simulink model "EMPlanner_850_155633_cs"  (R2023a)
settings: Solver=ode5  StartTime=0.0  StopTime=30  FixedStep=1/1000  RelTol=1e-3
PreLoadFcn:
  | mbxruntime.callbacks.PreLoadFcn(bdroot);
PostLoadFcn:
  | mbxruntime.callbacks.PostLoadFcn(bdroot);
InitFcn:
  | mbxruntime.callbacks.InitFcn(bdroot);
StartFcn:
  | mbxruntime.callbacks.StartFcn(bdroot);
StopFcn:
  | mbxruntime.callbacks.StopFcn(bdroot);
model workspace (MAT data in the model file):
  mbox_table : object (value not decoded)
  model_closed = 0
  sim_status = 0
undefined symbols (not defined in the file): aubr, c_factor, cf, cr, DiscIntNeverNeededParam, global_path_x, global_path_y, KD_PID_distance, KD_PID_speed, KI_PID_distance, KI_PID_speed, KP_PID_distance, KP_PID_speed, la, lb, LQR_K1, LQR_K2, LQR_K3, LQR_K4, m, rack_displacement, right_wheel_ground, tablebr, vubr, vx_break_point, warningInitialVelocity, x0
libraries: PreScanSimulinkLibrary x39, simulink x19, simulink_extras x11, Solver_SF x1
(part 9 of 11)

== matlab function EMPlanner_850_155633_cs/Audi_A8_Sedan_1/decision&planning module/referenceline provider/MATLAB Function5 ==
  data: x_set input; match_point_index_set output; y_set input; frenet_path_x input; frenet_path_y input; frenet_path_heading input; frenet_path_kappa input; proj_x_set output; proj_y_set output; proj_heading_set output; proj_kappa_set output
function [match_point_index_set,proj_x_set, proj_y_set,proj_heading_set,proj_kappa_set] = ...
    fcn(x_set,y_set,frenet_path_x,frenet_path_y,frenet_path_heading,frenet_path_kappa)
%该函数将批量计算x_set，y_set中的xy，在frenet_path下的投影的信息
%输入 x_set,y_set，待投影的点的集合
%x_set,y_set,frenet_path_x,frenet_path_y,frenet_path_heading,frenet_path_kappa
%曲线在直角坐标系下的x，y，heading，kappa
%输出：match_point_index_set 匹配点在frenet_path下的编号的集合(即从全局路径第一个点开始数，第几个点是匹配点)
%     proj_x y heading kappa 投影的x,y,heading,kappa的集合

% 由于事先不知道x_set中到底有多少个点需要投影，因此事先声明一个最大的数量的点作为缓冲
n = 128;
% 并且由于不知道投影点的个数，所以也不知道输出的个数，因此输出也要做缓冲，用nan表示不存在的点
% 输出最多输出128个
% 输出初始化
match_point_index_set = ones(n,1) * nan;
proj_x_set = ones(n,1) * nan;
proj_y_set = ones(n,1) * nan;
proj_heading_set = ones(n,1) * nan;
proj_kappa_set = ones(n,1) * nan;

% 找匹配点，需要利用上一个周期的结果作为下一个周期遍历的起点，因此需要声明两个全局变量

persistent is_first_run;
persistent pre_match_point_index_set;%bug :pre_match_point_index(i) 未必代表的是第i个障碍物的match_point_index
persistent pre_frenet_path_x;
persistent pre_frenet_path_y;
persistent pre_frenet_path_heading;
persistent pre_frenet_path_kappa;
persistent pre_x_set;
persistent pre_y_set;
%算法主函数入口

if isempty(is_first_run)
    %该if分支表示函数首次运行
    is_first_run = 0;
    pre_frenet_path_x = frenet_path_x;
    pre_frenet_path_y = frenet_path_y;
    pre_frenet_path_heading = frenet_path_heading;
    pre_frenet_path_kappa = frenet_path_kappa;
    %要记录首次运行计算的匹配点的结果供下个周期运行，先初始化
    pre_match_point_index_set = ones(n,1) * nan;
    %对x_set,y_set的点做遍历，找到他们的匹配点
    for i = 1 : length(x_set)
        if isnan(x_set(i))
            break;
        end
        %首次运行时，没有任何提示，只能从frenet path的第一个点开始找
        start_search_index = 1;
        % 声明increase_count，用于表示在遍历时distance连续增加的个数
        increase_count = 0;
        % 开始遍历
        min_distance = inf;
        for j = start_search_index : length(frenet_path_x)
            distance = (x_set(i) - frenet_path_x(j))^2 + (y_set(i) - frenet_path_y(j))^2;
            if distance < min_distance
                min_distance = distance;
                match_point_index_set(i) = j;
                increase_count = 0;
            else
                increase_count = increase_count + 1;
            end
            %如果distance连续增加50次就不要再遍历了，节省时间
            if increase_count > 50
                break;
            end
        end
        
        %如何通过匹配点计算投影点，请参见《自动驾驶控制算法第七讲》
        %或《自动驾驶决策规划算法》第一章第三节
        
        %取出匹配点的编号
        match_point_index = match_point_index_set(i);
        %取出匹配点的信息
        match_point_x = frenet_path_x(match_point_index);
        match_point_y = frenet_path_y(match_point_index);
        match_point_heading = frenet_path_heading(match_point_index);
        match_point_kappa = frenet_path_kappa(match_point_index);
        %计算匹配点的方向向量与法向量
        vector_match_point = [match_point_x;match_point_y];
        vector_match_point_direction = [cos(match_point_heading);sin(match_point_heading)];
        %声明待投影点的位矢
        vector_r = [x_set(i);y_set(i)];
        
       %通过匹配点计算投影点
       vector_d = vector_r - vector_match_point;
       ds = vector_d' * vector_match_point_direction;
       vector_proj_point = vector_match_point + ds * vector_match_point_direction;
       proj_heading = match_point_heading + match_point_kappa * ds;
       proj_kappa = match_point_kappa;
       %计算结果输出
       proj_x_set(i) = vector_proj_point(1);
       proj_y_set(i) = vector_proj_point(2);
       proj_heading_set(i) = proj_heading;
       proj_kappa_set(i) = proj_kappa;
    end
    %匹配点的计算结果保存，供下一个周期使用
    pre_match_point_index_set = match_point_index_set;
    pre_x_set = x_set;
    pre_y_set = y_set;
else
    %此if分支表示不是首次运行
    %对每个x_set上的点做处理
    for i = 1 : length(x_set)
        %不是首次运行，对于点x_set(i),y_set(i)来说,start_search_index =
        %pre_match_point_index_set(i)
        start_search_index = pre_match_point_index_set(i);%上个周期匹配点的编号作为本周期搜索的起点
        % 判断帧与帧之间的障碍物是否为同一个
        square_dis = (x_set(i) - pre_x_set(i))^2 + (y_set(i) - pre_y_set(i))^2;
        if square_dis > 36
            % 帧与帧之间的物体的位置距离过大，认为是两个障碍物
            start_search_index = nan;
        end
        % 声明increase_count，用于表示在遍历时distance连续增加的个数
        %%%%%%%%%
        %对于障碍物检测而言，当感知第一次检测到障碍物时，算法并不是首次运行，此时 
        %pre_match_point_index_set的值是nan，如果还用上一时刻的结果作为本周期搜索的起点
        %必然会出问题，所以要修改
        % 声明increase_count_limit
        increase_count_limit = 5;
        if isnan(start_search_index)
            %没有上个周期的结果，那就不能只检查5次了
            increase_count_limit = 50;
            %搜索起点也要设为1
            start_search_index = 1;
        end
        increase_count = 0;
        % 开始遍历
        %这里多一个步骤，判断遍历的方向
        %计算上个周期匹配点的位矢
        vector_pre_match_point = [pre_frenet_path_x(start_search_index);pre_frenet_path_y(start_search_index)];
        vector_pre_match_point_direction = ...
            [cos(pre_frenet_path_heading(start_search_index));sin(pre_frenet_path_heading(start_search_index))];
        %判断遍历的方向
        flag = ([x_set(i);y_set(i)] - vector_pre_match_point)' * vector_pre_match_point_direction;
        min_distance = inf;
        if flag > 0.001
            for j = start_search_index : length(frenet_path_x)
                distance = (x_set(i) - frenet_path_x(j))^2 + (y_set(i) - frenet_path_y(j))^2;
                if distance < min_distance
                    min_distance = distance;
                    match_point_index_set(i) = j;
                    increase_count = 0;
                else
                    increase_count = increase_count + 1;
                end
                %如果distance连续增加increase_count_limit次就不要再遍历了，节省时间
                if increase_count > increase_count_limit
                    break;
                end
            end
        elseif flag < - 0.001
            for j = start_search_index : -1 : 1
                distance = (x_set(i) - frenet_path_x(j))^2 + (y_set(i) - frenet_path_y(j))^2;
                if distance < min_distance
                    min_distance = distance;
                    match_point_index_set(i) = j;
                    increase_count = 0;
                else
                    increase_count = increase_count + 1;
                end
                %如果distance连续增加increase_count_limit次就不要再遍历了，节省时间
                if increase_count > increase_count_limit
                    break;
                end
            end
        else
            match_point_index_set(i) = start_search_index;
        end
        
        %如何通过匹配点计算投影点，请参见《自动驾驶控制算法第七讲》
        %或《自动驾驶决策规划算法》第一章第三节
        
        %取出匹配点的编号
        match_point_index = match_point_index_set(i);
        %取出匹配点的信息
        match_point_x = frenet_path_x(match_point_index);
        match_point_y = frenet_path_y(match_point_index);
        match_point_heading = frenet_path_heading(match_point_index);
        match_point_kappa = frenet_path_kappa(match_point_index);
        %计算匹配点的方向向量与法向量
        vector_match_point = [match_point_x;match_point_y];
        vector_match_point_direction = [cos(match_point_heading);sin(match_point_heading)];
        %声明待投影点的位矢
        vector_r = [x_set(i);y_set(i)];
        
       %通过匹配点计算投影点
       vector_d = vector_r - vector_match_point;
       ds = vector_d' * vector_match_point_direction;
       vector_proj_point = vector_match_point + ds * vector_match_point_direction;
       proj_heading = match_point_heading + match_point_kappa * ds;
       proj_kappa = match_point_kappa;
       %计算结果输出
       proj_x_set(i) = vector_proj_point(1);
       proj_y_set(i) = vector_proj_point(2);
       proj_heading_set(i) = proj_heading;
       proj_kappa_set(i) = proj_kappa;
  
    end
    %匹配点的计算结果保存，供下一个周期使用
    pre_match_point_index_set = match_point_index_set;
    pre_frenet_path_x = frenet_path_x;
    pre_frenet_path_y = frenet_path_y;
    pre_frenet_path_heading = frenet_path_heading;
    pre_frenet_path_kappa = frenet_path_kappa;
    pre_x_set = x_set;
    pre_y_set = y_set;
end

== matlab function EMPlanner_850_155633_cs/Audi_A8_Sedan_1/decision&planning module/EM Planner/genrate index to s ==
  data: path_x input; index2s output; path_y input; origin_x input; origin_y input; origin_match_point_index input
function index2s  = fcn(path_x,path_y,origin_x,origin_y,origin_match_point_index)
%该函数将输出index与s的转换关系，index2s表示当path_x,path_y的离散点的编号为i时，对应的弧长为index2s(i)
%输入 path_x path_y 待转化的离散点的集合
%     origin_x,y frenet原点在世界坐标系下的坐标
%     origin_match_point_index 原点的匹配点的编号
% path点的个数
n = 181;
% 输出初始化
index2s = zeros(n,1);
% 首先计算以path起点为坐标原点的index2s
for i = 2:n
    index2s(i) = sqrt((path_x(i) - path_x(i-1))^2 + (path_y(i) - path_y(i-1))^2) + index2s(i-1);
end
% 再计算以轨迹起点到frenet_path的坐标原点的弧长，记为s0，再用index2s - s0 就是最终的结果
% 计算s0
% s_temp frenet原点的匹配点的弧长
s_temp = index2s(origin_match_point_index);
%判断原点在匹配点的前面还是后面
%两个向量match_point_to_origin 
%        match_point_to_match_point_next
vector_match_2_origin = [origin_x;origin_y] - [path_x(origin_match_point_index);path_y(origin_match_point_index)];
vector_match_2_match_next = [path_x(origin_match_point_index + 1);path_y(origin_match_point_index + 1)] - ...
                            [path_x(origin_match_point_index);path_y(origin_match_point_index)];
if vector_match_2_origin'*vector_match_2_match_next > 0
    %坐标原点在匹配点的前面
    s0 = s_temp + sqrt(vector_match_2_origin'*vector_match_2_origin);
else
    %坐标原点在匹配点的后面
    s0 = s_temp - sqrt(vector_match_2_origin'*vector_match_2_origin);
end

index2s = index2s - ones(n,1)*s0;

== stateflow chart EMPlanner_850_155633_cs/Audi_A8_Sedan_1/Chart ==
  (default) -> (junction 5)
  (junction 5) -> (junction 7)
  (junction 7) -> (junction 9) [order 1] : [i >= 100]
  (junction 7) -> (junction 13) [order 2] : {
      | i = i + 1;
      | }
  (junction 9) -> (junction 11) : {
      | do_planning;
      | i = 1;
      | }
  (junction 11) -> (junction 13)
  (junction 13) -> (junction 16)
  (junction 16) -> (junction 18) [order 1] : [j >= 10]
  (junction 16) -> (junction 22) [order 2] : {
      | j = j + 1;
      | }
  (junction 18) -> (junction 20) : {
      | do_control;
      | j = 1;
      | }
  (junction 20) -> (junction 22)
  (junction 22) -> (junction 25)
  data: i local =1; j local =1
  events: do_planning output FUNCTION_CALL_EVENT; do_control output FUNCTION_CALL_EVENT

== matlab function EMPlanner_850_155633_cs/Audi_A8_Sedan_1/decision&planning module/referenceline provider/MATLAB Function6 ==
  data: x_set input; match_point_index_set output; y_set input; frenet_path_x input; frenet_path_y input; frenet_path_heading input; frenet_path_kappa input; proj_x_set output; proj_y_set output; proj_heading_set output; proj_kappa_set output
function [match_point_index_set,proj_x_set, proj_y_set,proj_heading_set,proj_kappa_set] = ...
    fcn(x_set,y_set,frenet_path_x,frenet_path_y,frenet_path_heading,frenet_path_kappa)
%该函数将批量计算x_set，y_set中的xy，在frenet_path下的投影的信息
%输入 x_set,y_set，待投影的点的集合
%x_set,y_set,frenet_path_x,frenet_path_y,frenet_path_heading,frenet_path_kappa
%曲线在直角坐标系下的x，y，heading，kappa
%输出：match_point_index_set 匹配点在frenet_path下的编号的集合(即从全局路径第一个点开始数，第几个点是匹配点)
%     proj_x y heading kappa 投影的x,y,heading,kappa的集合

% 由于事先不知道x_set中到底有多少个点需要投影，因此事先声明一个最大的数量的点作为缓冲
n = 128;
% 并且由于不知道投影点的个数，所以也不知道输出的个数，因此输出也要做缓冲，用nan表示不存在的点
% 输出最多输出128个
% 输出初始化
match_point_index_set = ones(n,1) * nan;
proj_x_set = ones(n,1) * nan;
proj_y_set = ones(n,1) * nan;
proj_heading_set = ones(n,1) * nan;
proj_kappa_set = ones(n,1) * nan;

% 找匹配点，需要利用上一个周期的结果作为下一个周期遍历的起点，因此需要声明两个全局变量

persistent is_first_run;
persistent pre_match_point_index_set;%bug :pre_match_point_index(i) 未必代表的是第i个障碍物的match_point_index
persistent pre_frenet_path_x;
persistent pre_frenet_path_y;
persistent pre_frenet_path_heading;
persistent pre_frenet_path_kappa;
persistent pre_x_set;
persistent pre_y_set;
%算法主函数入口

if isempty(is_first_run)
    %该if分支表示函数首次运行
    is_first_run = 0;
    pre_frenet_path_x = frenet_path_x;
    pre_frenet_path_y = frenet_path_y;
    pre_frenet_path_heading = frenet_path_heading;
    pre_frenet_path_kappa = frenet_path_kappa;
    %要记录首次运行计算的匹配点的结果供下个周期运行，先初始化
    pre_match_point_index_set = ones(n,1) * nan;
    %对x_set,y_set的点做遍历，找到他们的匹配点
    for i = 1 : length(x_set)
        if isnan(x_set(i))
            break;
        end
        %首次运行时，没有任何提示，只能从frenet path的第一个点开始找
        start_search_index = 1;
        % 声明increase_count，用于表示在遍历时distance连续增加的个数
        increase_count = 0;
        % 开始遍历
        min_distance = inf;
        for j = start_search_index : length(frenet_path_x)
            distance = (x_set(i) - frenet_path_x(j))^2 + (y_set(i) - frenet_path_y(j))^2;
            if distance < min_distance
                min_distance = distance;
                match_point_index_set(i) = j;
                increase_count = 0;
            else
                increase_count = increase_count + 1;
            end
            %如果distance连续增加50次就不要再遍历了，节省时间
            if increase_count > 50
                break;
            end
        end
        
        %如何通过匹配点计算投影点，请参见《自动驾驶控制算法第七讲》
        %或《自动驾驶决策规划算法》第一章第三节
        
        %取出匹配点的编号
        match_point_index = match_point_index_set(i);
        %取出匹配点的信息
        match_point_x = frenet_path_x(match_point_index);
        match_point_y = frenet_path_y(match_point_index);
        match_point_heading = frenet_path_heading(match_point_index);
        match_point_kappa = frenet_path_kappa(match_point_index);
        %计算匹配点的方向向量与法向量
        vector_match_point = [match_point_x;match_point_y];
        vector_match_point_direction = [cos(match_point_heading);sin(match_point_heading)];
        %声明待投影点的位矢
        vector_r = [x_set(i);y_set(i)];
        
       %通过匹配点计算投影点
       vector_d = vector_r - vector_match_point;
       ds = vector_d' * vector_match_point_direction;
       vector_proj_point = vector_match_point + ds * vector_match_point_direction;
       proj_heading = match_point_heading + match_point_kappa * ds;
       proj_kappa = match_point_kappa;
       %计算结果输出
       proj_x_set(i) = vector_proj_point(1);
       proj_y_set(i) = vector_proj_point(2);
       proj_heading_set(i) = proj_heading;
       proj_kappa_set(i) = proj_kappa;
    end
    %匹配点的计算结果保存，供下一个周期使用
    pre_match_point_index_set = match_point_index_set;
    pre_x_set = x_set;
    pre_y_set = y_set;
else
    %此if分支表示不是首次运行
    %对每个x_set上的点做处理
    for i = 1 : length(x_set)
        %不是首次运行，对于点x_set(i),y_set(i)来说,start_search_index =
        %pre_match_point_index_set(i)
        start_search_index = pre_match_point_index_set(i);%上个周期匹配点的编号作为本周期搜索的起点
        % 判断帧与帧之间的障碍物是否为同一个
        square_dis = (x_set(i) - pre_x_set(i))^2 + (y_set(i) - pre_y_set(i))^2;
        if square_dis > 36
            % 帧与帧之间的物体的位置距离过大，认为是两个障碍物
            start_search_index = nan;
        end
        % 声明increase_count，用于表示在遍历时distance连续增加的个数
        %%%%%%%%%
        %对于障碍物检测而言，当感知第一次检测到障碍物时，算法并不是首次运行，此时 
        %pre_match_point_index_set的值是nan，如果还用上一时刻的结果作为本周期搜索的起点
        %必然会出问题，所以要修改
        % 声明increase_count_limit
        increase_count_limit = 5;
        if isnan(start_search_index)
            %没有上个周期的结果，那就不能只检查5次了
            increase_count_limit = 50;
            %搜索起点也要设为1
            start_search_index = 1;
        end
        increase_count = 0;
        % 开始遍历
        %这里多一个步骤，判断遍历的方向
        %计算上个周期匹配点的位矢
        vector_pre_match_point = [pre_frenet_path_x(start_search_index);pre_frenet_path_y(start_search_index)];
        vector_pre_match_point_direction = ...
            [cos(pre_frenet_path_heading(start_search_index));sin(pre_frenet_path_heading(start_search_index))];
        %判断遍历的方向
        flag = ([x_set(i);y_set(i)] - vector_pre_match_point)' * vector_pre_match_point_direction;
        min_distance = inf;
        if flag > 0.001
            for j = start_search_index : length(frenet_path_x)
                distance = (x_set(i) - frenet_path_x(j))^2 + (y_set(i) - frenet_path_y(j))^2;
                if distance < min_distance
                    min_distance = distance;
                    match_point_index_set(i) = j;
                    increase_count = 0;
                else
                    increase_count = increase_count + 1;
                end
                %如果distance连续增加increase_count_limit次就不要再遍历了，节省时间
                if increase_count > increase_count_limit
                    break;
                end
            end
        elseif flag < - 0.001
            for j = start_search_index : -1 : 1
                distance = (x_set(i) - frenet_path_x(j))^2 + (y_set(i) - frenet_path_y(j))^2;
                if distance < min_distance
                    min_distance = distance;
                    match_point_index_set(i) = j;
                    increase_count = 0;
                else
                    increase_count = increase_count + 1;
                end
                %如果distance连续增加increase_count_limit次就不要再遍历了，节省时间
                if increase_count > increase_count_limit
                    break;
                end
            end
        else
            match_point_index_set(i) = start_search_index;
        end
        
        %如何通过匹配点计算投影点，请参见《自动驾驶控制算法第七讲》
        %或《自动驾驶决策规划算法》第一章第三节
        
        %取出匹配点的编号
        match_point_index = match_point_index_set(i);
        %取出匹配点的信息
        match_point_x = frenet_path_x(match_point_index);
        match_point_y = frenet_path_y(match_point_index);
        match_point_heading = frenet_path_heading(match_point_index);
        match_point_kappa = frenet_path_kappa(match_point_index);
        %计算匹配点的方向向量与法向量
        vector_match_point = [match_point_x;match_point_y];
        vector_match_point_direction = [cos(match_point_heading);sin(match_point_heading)];
        %声明待投影点的位矢
        vector_r = [x_set(i);y_set(i)];
        
       %通过匹配点计算投影点
       vector_d = vector_r - vector_match_point;
       ds = vector_d' * vector_match_point_direction;
       vector_proj_point = vector_match_point + ds * vector_match_point_direction;
       proj_heading = match_point_heading + match_point_kappa * ds;
       proj_kappa = match_point_kappa;
       %计算结果输出
       proj_x_set(i) = vector_proj_point(1);
       proj_y_set(i) = vector_proj_point(2);
       proj_heading_set(i) = proj_heading;
       proj_kappa_set(i) = proj_kappa;
  
    end
    %匹配点的计算结果保存，供下一个周期使用
    pre_match_point_index_set = match_point_index_set;
    pre_frenet_path_x = frenet_path_x;
    pre_frenet_path_y = frenet_path_y;
    pre_frenet_path_heading = frenet_path_heading;
    pre_frenet_path_kappa = frenet_path_kappa;
    pre_x_set = x_set;
    pre_y_set = y_set;
end

== matlab function EMPlanner_850_155633_cs/Audi_A8_Sedan_1/decision&planning module/EM Planner/Cartesian2Frenet/MATLAB Function ==
  data: x_set input; s_set output; y_set input; frenet_path_x input; frenet_path_y input; proj_x_set input; proj_y_set input; proj_heading_set input; proj_match_point_index_set input; index2s input; l_set output
function [s_set,l_set] = fcn(x_set,y_set,frenet_path_x,frenet_path_y,...
    proj_x_set,proj_y_set,proj_heading_set,proj_match_point_index_set,index2s)
    %该函数将计算世界坐标系下的x_set，y_set上的点在frenet_path下的坐标s l
    %输入 x_set,y_set 待坐标转换的点
    %     frenet_path_x,frenet_path_y   frenet坐标轴
    %     proj_x,y,heading,kappa,proj_match_point_index 待坐标转换的点的投影点的信息
    %     index2s   frenet_path的index与s的转换表

    % 由于不知道有多少个点需要做坐标转换，所以需要做缓冲
    n = 128;%最多处理128个点
    %输出初始化
    s_set = ones(n,1)*nan;
    l_set = ones(n,1)*nan;
    for i = 1:length(x_set)
        if isnan(x_set(i))
            break;
        end
        %计算s，写个子函数
        s_set(i) = CalcSFromIndex2S(index2s,frenet_path_x,frenet_path_y,proj_x_set(i),proj_y_set(i),...
            proj_match_point_index_set(i));
        n_r = [-sin(proj_heading_set(i));cos(proj_heading_set(i))];
        r_h = [x_set(i);y_set(i)];
        r_r = [proj_x_set(i);proj_y_set(i)];
        l_set(i) = (r_h - r_r)'*n_r;
    end
end

function s = CalcSFromIndex2S(index2s,path_x,path_y,proj_x,proj_y,proj_match_point_index)
  %该函数将计算当指定index2s的映射关系后，计算点proj_x,proj_y的弧长
  vector_1 = [proj_x;proj_y] - [path_x(proj_match_point_index);path_y(proj_match_point_index)];
  %这里要考虑的更全面一些，因为要考虑到proj_match_point_index有可能在path的起点或终点
  if (proj_match_point_index < length(path_x))
      vector_2 = [path_x(proj_match_point_index + 1);path_y(proj_match_point_index + 1)] - ...
          [path_x(proj_match_point_index);path_y(proj_match_point_index)];
  else
      vector_2 = [path_x(proj_match_point_index);path_y(proj_match_point_index)] - ...
          [path_x(proj_match_point_index - 1);path_y(proj_match_point_index - 1)];
  end
  
  if vector_1'*vector_2 > 0
      s = index2s(proj_match_point_index) + sqrt(vector_1'*vector_1);
  else
      s = index2s(proj_match_point_index) - sqrt(vector_1'*vector_1);
  end
  
  
end

== matlab function EMPlanner_850_155633_cs/Audi_A8_Sedan_1/control module1/control main/chassic steering system/MATLAB Function ==
  data: u input; right_steer output; la input; lb input
function right_steer = fcn(u,la,lb)
if abs(u)<1e-2
   right_steer = u;
else
   R =  (la+lb)/tan(u);
   right_steer = atan((la+lb)/(R+1.624/2));
end

== matlab function EMPlanner_850_155633_cs/Audi_A8_Sedan_1/control module1/control main/lateral control LQR/calc lqr K ==
  data: k1 input; k output; k2 input; k3 input; k4 input; vx input
function k  = fcn(k1,k2,k3,k4,vx)
    if abs(vx)<0.1
        k=[0,0,0,0];
    else
       
        k=[k1,k2,k3,k4];
    end
end

== matlab function EMPlanner_850_155633_cs/Audi_A8_Sedan_1/control module1/control main/lateral control LQR/err_kappa_calculate_module ==
  data: x input; y input; phi input; vx input; vy input; phi_dot input; xr input; yr input; thetar input; kappar input; err output; es output; s_dot output; phi output; projection_point_thetar output
function [err,es,s_dot,phi,projection_point_thetar] = fcn(x,y,phi,vx,vy,phi_dot,xr,yr,thetar,kappar)
    
    tor=[cos(thetar);sin(thetar)];
    nor=[-sin(thetar);cos(thetar)];
    d_err=[x-xr;y-yr];
    ed=nor'*d_err;
    es=tor'*d_err;
    %projection_point_thetar=thetar(dmin);%apollo
    projection_point_thetar=thetar+kappar*es;
    ed_dot=vy*cos(phi-projection_point_thetar)+vx*sin(phi-projection_point_thetar);
    %%%%%%%%%
    ephi=sin(phi-projection_point_thetar);
    %%%%%%%%%
    ss_dot=vx*cos(phi-projection_point_thetar)-vy*sin(phi-projection_point_thetar);
    s_dot=ss_dot/(1-kappar*ed);
    ephi_dot=phi_dot-kappar*s_dot;
    err=[ed;ed_dot;ephi;ephi_dot];
    
    
    
    
    
    
    
    
    
    
    
    


end

== matlab function EMPlanner_850_155633_cs/Audi_A8_Sedan_1/control module1/control main/lateral control LQR/feed_forword_control ==
  data: vx input; a input; forword_angle output; b input; m input; cf input; cr input; k input; kr input
function forword_angle = fcn(vx,a,b,m,cf,cr,k,kr)
    forword_angle=kr*(a+b-b*k(3)-(m*vx*vx/(a+b))*((b/cf)+(a/cr)*k(3)-(a/cr)));
end

== matlab function EMPlanner_850_155633_cs/Audi_A8_Sedan_1/control module1/control main/lateral control LQR/feedback_control+feedforword_control ==
  data: k input; angle output; err input; forword_angle input
function angle = fcn(k,err,forword_angle)

    angle=-k*err+forword_angle;
end

== matlab function EMPlanner_850_155633_cs/Audi_A8_Sedan_1/control module1/control main/lateral control LQR/predict_module ==
  data: x input; pred_x_ctrl output; y input; phi input; vx input; vy input; phi_dot input; ts input; pred_y_ctrl output; pred_yaw_ctrl output; pred_vx_ctrl output; pred_vy_ctrl output; pred_yaw_dot_ctrl output
function [pred_x_ctrl,pred_y_ctrl,pred_yaw_ctrl,pred_vx_ctrl,pred_vy_ctrl,pred_yaw_dot_ctrl] = fcn(x,y,phi,vx,vy,phi_dot,ts)
    pred_x_ctrl=x+vx*ts*cos(phi)-vy*ts*sin(phi);
    pred_y_ctrl=y+vy*ts*cos(phi)+vx*ts*sin(phi);
    pred_yaw_ctrl=phi;
    pred_vx_ctrl=vx;
    pred_vy_ctrl=vy;
    pred_yaw_dot_ctrl=phi_dot;
end

== matlab function EMPlanner_850_155633_cs/Audi_A8_Sedan_1/control module1/control main/longitudinal control double PID/MATLAB Function1 ==
  data: u input; throttle output; brake output
function [throttle,brake] = fcn(u)
    if u>=0
        throttle=u;
        brake=0;
    else
        throttle=0;
        brake=-u;
    end

== matlab function EMPlanner_850_155633_cs/Audi_A8_Sedan_1/decision&planning module/EM Planner/obs/MATLAB Function2 ==
  data: x_set input; match_point_index_set output; y_set input; frenet_path_x input; frenet_path_y input; frenet_path_heading input; frenet_path_kappa input; proj_x_set output; proj_y_set output; proj_heading_set output; proj_kappa_set output
function [match_point_index_set,proj_x_set, proj_y_set,proj_heading_set,proj_kappa_set] = ...
    fcn(x_set,y_set,frenet_path_x,frenet_path_y,frenet_path_heading,frenet_path_kappa)
%该函数将批量计算x_set，y_set中的xy，在frenet_path下的投影的信息
%输入 x_set,y_set，待投影的点的集合
%x_set,y_set,frenet_path_x,frenet_path_y,frenet_path_heading,frenet_path_kappa
%曲线在直角坐标系下的x，y，heading，kappa
%输出：match_point_index_set 匹配点在frenet_path下的编号的集合(即从全局路径第一个点开始数，第几个点是匹配点)
%     proj_x y heading kappa 投影的x,y,heading,kappa的集合

% 由于事先不知道x_set中到底有多少个点需要投影，因此事先声明一个最大的数量的点作为缓冲
n = 128;
% 并且由于不知道投影点的个数，所以也不知道输出的个数，因此输出也要做缓冲，用nan表示不存在的点
% 输出最多输出128个
% 输出初始化
match_point_index_set = ones(n,1) * nan;
proj_x_set = ones(n,1) * nan;
proj_y_set = ones(n,1) * nan;
proj_heading_set = ones(n,1) * nan;
proj_kappa_set = ones(n,1) * nan;

% 找匹配点，需要利用上一个周期的结果作为下一个周期遍历的起点，因此需要声明两个全局变量

persistent is_first_run;
persistent pre_match_point_index_set;%bug :pre_match_point_index(i) 未必代表的是第i个障碍物的match_point_index
persistent pre_frenet_path_x;
persistent pre_frenet_path_y;
persistent pre_frenet_path_heading;
persistent pre_frenet_path_kappa;
persistent pre_x_set;
persistent pre_y_set;
%算法主函数入口

if isempty(is_first_run)
    %该if分支表示函数首次运行
    is_first_run = 0;
    pre_frenet_path_x = frenet_path_x;
    pre_frenet_path_y = frenet_path_y;
    pre_frenet_path_heading = frenet_path_heading;
    pre_frenet_path_kappa = frenet_path_kappa;
    %要记录首次运行计算的匹配点的结果供下个周期运行，先初始化
    pre_match_point_index_set = ones(n,1) * nan;
    %对x_set,y_set的点做遍历，找到他们的匹配点
    for i = 1 : length(x_set)
        if isnan(x_set(i))
            break;
        end
        %首次运行时，没有任何提示，只能从frenet path的第一个点开始找
        start_search_index = 1;
        % 声明increase_count，用于表示在遍历时distance连续增加的个数
        increase_count = 0;
        % 开始遍历
        min_distance = inf;
        for j = start_search_index : length(frenet_path_x)
            distance = (x_set(i) - frenet_path_x(j))^2 + (y_set(i) - frenet_path_y(j))^2;
            if distance < min_distance
                min_distance = distance;
                match_point_index_set(i) = j;
                increase_count = 0;
            else
                increase_count = increase_count + 1;
            end
            %如果distance连续增加50次就不要再遍历了，节省时间
            if increase_count > 50
                break;
            end
        end
        
        %如何通过匹配点计算投影点，请参见《自动驾驶控制算法第七讲》
        %或《自动驾驶决策规划算法》第一章第三节
        
        %取出匹配点的编号
        match_point_index = match_point_index_set(i);
        %取出匹配点的信息
        match_point_x = frenet_path_x(match_point_index);
        match_point_y = frenet_path_y(match_point_index);
        match_point_heading = frenet_path_heading(match_point_index);
        match_point_kappa = frenet_path_kappa(match_point_index);
        %计算匹配点的方向向量与法向量
        vector_match_point = [match_point_x;match_point_y];
        vector_match_point_direction = [cos(match_point_heading);sin(match_point_heading)];
        %声明待投影点的位矢
        vector_r = [x_set(i);y_set(i)];
        
       %通过匹配点计算投影点
       vector_d = vector_r - vector_match_point;
       ds = vector_d' * vector_match_point_direction;
       vector_proj_point = vector_match_point + ds * vector_match_point_direction;
       proj_heading = match_point_heading + match_point_kappa * ds;
       proj_kappa = match_point_kappa;
       %计算结果输出
       proj_x_set(i) = vector_proj_point(1);
       proj_y_set(i) = vector_proj_point(2);
       proj_heading_set(i) = proj_heading;
       proj_kappa_set(i) = proj_kappa;
    end
    %匹配点的计算结果保存，供下一个周期使用
    pre_match_point_index_set = match_point_index_set;
    pre_x_set = x_set;
    pre_y_set = y_set;
else
    %此if分支表示不是首次运行
    %对每个x_set上的点做处理
    for i = 1 : length(x_set)
        %不是首次运行，对于点x_set(i),y_set(i)来说,start_search_index =
        %pre_match_point_index_set(i)
        start_search_index = pre_match_point_index_set(i);%上个周期匹配点的编号作为本周期搜索的起点
        % 判断帧与帧之间的障碍物是否为同一个
        square_dis = (x_set(i) - pre_x_set(i))^2 + (y_set(i) - pre_y_set(i))^2;
        if square_dis > 36
            % 帧与帧之间的物体的位置距离过大，认为是两个障碍物
            start_search_index = nan;
        end
        % 声明increase_count，用于表示在遍历时distance连续增加的个数
        %%%%%%%%%
        %对于障碍物检测而言，当感知第一次检测到障碍物时，算法并不是首次运行，此时 
        %pre_match_point_index_set的值是nan，如果还用上一时刻的结果作为本周期搜索的起点
        %必然会出问题，所以要修改
        % 声明increase_count_limit
        increase_count_limit = 5;
        if isnan(start_search_index)
            %没有上个周期的结果，那就不能只检查5次了
            increase_count_limit = 50;
            %搜索起点也要设为1
            start_search_index = 1;
        end
        increase_count = 0;
        % 开始遍历
        %这里多一个步骤，判断遍历的方向
        %计算上个周期匹配点的位矢
        vector_pre_match_point = [pre_frenet_path_x(start_search_index);pre_frenet_path_y(start_search_index)];
        vector_pre_match_point_direction = ...
            [cos(pre_frenet_path_heading(start_search_index));sin(pre_frenet_path_heading(start_search_index))];
        %判断遍历的方向
        flag = ([x_set(i);y_set(i)] - vector_pre_match_point)' * vector_pre_match_point_direction;
        min_distance = inf;
        if flag > 0.001
            for j = start_search_index : length(frenet_path_x)
                distance = (x_set(i) - frenet_path_x(j))^2 + (y_set(i) - frenet_path_y(j))^2;
                if distance < min_distance
                    min_distance = distance;
                    match_point_index_set(i) = j;
                    increase_count = 0;
                else
                    increase_count = increase_count + 1;
                end
                %如果distance连续增加increase_count_limit次就不要再遍历了，节省时间
                if increase_count > increase_count_limit
                    break;
                end
            end
        elseif flag < - 0.001
            for j = start_search_index : -1 : 1
                distance = (x_set(i) - frenet_path_x(j))^2 + (y_set(i) - frenet_path_y(j))^2;
                if distance < min_distance
                    min_distance = distance;
                    match_point_index_set(i) = j;
                    increase_count = 0;
                else
                    increase_count = increase_count + 1;
                end
                %如果distance连续增加increase_count_limit次就不要再遍历了，节省时间
                if increase_count > increase_count_limit
                    break;
                end
            end
        else
            match_point_index_set(i) = start_search_index;
        end
        
        %如何通过匹配点计算投影点，请参见《自动驾驶控制算法第七讲》
        %或《自动驾驶决策规划算法》第一章第三节
        
        %取出匹配点的编号
        match_point_index = match_point_index_set(i);
        %取出匹配点的信息
        match_point_x = frenet_path_x(match_point_index);
        match_point_y = frenet_path_y(match_point_index);
        match_point_heading = frenet_path_heading(match_point_index);
        match_point_kappa = frenet_path_kappa(match_point_index);
        %计算匹配点的方向向量与法向量
        vector_match_point = [match_point_x;match_point_y];
        vector_match_point_direction = [cos(match_point_heading);sin(match_point_heading)];
        %声明待投影点的位矢
        vector_r = [x_set(i);y_set(i)];
        
       %通过匹配点计算投影点
       vector_d = vector_r - vector_match_point;
       ds = vector_d' * vector_match_point_direction;
       vector_proj_point = vector_match_point + ds * vector_match_point_direction;
       proj_heading = match_point_heading + match_point_kappa * ds;
       proj_kappa = match_point_kappa;
       %计算结果输出
       proj_x_set(i) = vector_proj_point(1);
       proj_y_set(i) = vector_proj_point(2);
       proj_heading_set(i) = proj_heading;
       proj_kappa_set(i) = proj_kappa;
  
    end
    %匹配点的计算结果保存，供下一个周期使用
    pre_match_point_index_set = match_point_index_set;
    pre_frenet_path_x = frenet_path_x;
    pre_frenet_path_y = frenet_path_y;
    pre_frenet_path_heading = frenet_path_heading;
    pre_frenet_path_kappa = frenet_path_kappa;
    pre_x_set = x_set;
    pre_y_set = y_set;
end

== matlab function EMPlanner_850_155633_cs/Audi_A8_Sedan_1/decision&planning module/referenceline provider/MATLAB Function3 ==
  data: path_x input; path_heading output; path_y input; path_kappa output
function [path_heading,path_kappa] = fcn(path_x,path_y)
%该函数将计算path的切线方向与x轴的夹角和曲率
%输入：path_x,y路径坐标
%输出：path heading kappa 路径的heading和曲率
%原理 heading = arctan(dy/dx);
%     kappa = dheading/ds;
%     ds = (dx^2 + dy^2)^0.5

%注意，角度的多值性会带来很大的麻烦，需要慎重处理
%例，x 与 x + 2pi往往代表同一个角度，这种多值性在计算曲率会带来麻烦
%比如 原本是(0.1 - (-0.1))/ds，但如果计算出的-0.1多了一个2pi
%kappa就等于(0.1 - (-0.1 + 2*pi))/ds，曲率会变得非常大
%还有若采用中点欧拉法计算heading时，(即使用(y2 - y1)/(x2 - x1)的反正切计算一个角度 ，用(y1 - y0)/(x1
%-x0)的反正切又计算一个角度，然后加起来除以2),如果精确值是 (a1 + a2)/2,但最终计算的结果可能是(a1 + a2 + 2pi)/2
% 还有 tan(x) = tan(x + pi) 所以arctan(tan(x))可能等于x，也可能等于x + pi
% 角度的处理非常麻烦，而且角度处理不当往往是许多奇怪错误的源头

dx = diff(path_x);
dy = diff(path_y);
%用中点欧拉法要比向前欧拉法向后欧拉法更精确，但是也可能计算出的结果比精确值多一个pi
%在这里对dx,dy做中点欧拉法，使用四象限反正切计算角度
dx_pre = [dx(1);dx];
dx_after = [dx;dx(end)];
dx_final = (dx_pre + dx_after)/2;

dy_pre = [dy(1);dy];
dy_after = [dy;dy(end)];
dy_final = (dy_pre + dy_after)/2;

ds_final = sqrt(dx_final.^2 + dy_final.^2);
path_heading = atan2(dy_final,dx_final);

dheading = diff(path_heading);
dheading_pre = [dheading(1);dheading];
dheading_after = [dheading;dheading(end)];
dheading_final = (dheading_pre + dheading_after) / 2;
%为了防止dheading出现多一个2pi的错误，假设真实的dheading较小，用sin(dheading)近似dheading
path_kappa = sin(dheading_final) ./ ds_final;

== matlab function EMPlanner_850_155633_cs/Audi_A8_Sedan_1/decision&planning module/EM Planner/Cartesian2Frenet/MATLAB Function1 ==
  data: l_set input; s_dot_set output; vx_set input; vy_set input; proj_heading_set input; proj_kappa_set input; l_dot_set output; dl_set output
function [s_dot_set,l_dot_set,dl_set] = fcn(l_set,vx_set,vy_set,proj_heading_set,proj_kappa_set)
%该函数将计算frenet坐标系下的s_dot, l_dot, dl/ds
n = 128;
% 输出初始化
s_dot_set = ones(n,1)*nan;
l_dot_set = ones(n,1)*nan;
dl_set = ones(n,1)*nan;

for i = 1 : length(l_set)
    if isnan(l_set(i))
        break;
    end
    v_h = [vx_set(i);vy_set(i)];
    n_r = [-sin(proj_heading_set(i));cos(proj_heading_set(i))];
    t_r = [cos(proj_heading_set(i));sin(proj_heading_set(i))];
    l_dot_set(i) = v_h'*n_r;
    s_dot_set(i) = v_h'*t_r/(1 - proj_kappa_set(i)*l_set(i));
    %%%向量法做cartesian与frenet的转换要更简单，但是也有缺点，向量法必须依赖速度加速度
    %l' = l_dot/s_dot 但是如果s_dot = 0 此方法就失效了
    if abs(s_dot_set(i)) < 1e-6
        dl_set(i) = 0;
    else
        dl_set(i) = l_dot_set(i)/s_dot_set(i);
    end
end

== matlab function EMPlanner_850_155633_cs/Audi_A8_Sedan_1/decision&planning module/EM Planner/Cartesian2Frenet/MATLAB Function2 ==
  data: ax_set input; s_dot2_set output; ay_set input; proj_heading_set input; proj_kappa_set input; l_set input; s_dot_set input; dl_set input; l_dot2_set output; ddl_set output
function [s_dot2_set,l_dot2_set,ddl_set] = fcn(ax_set,ay_set,proj_heading_set,proj_kappa_set,l_set,s_dot_set,dl_set)
%由于不知道有多少个点需要做坐标转换，设一个最大值做缓冲
n = 128;
% 输出初始化
s_dot2_set = ones(n,1)*nan;
l_dot2_set = ones(n,1)*nan;
ddl_set = ones(n,1)*nan;

for i = 1:length(l_set)
    if isnan(l_set(i))
       break;
    end
    a_h = [ax_set(i);ay_set(i)];
    n_r = [-sin(proj_heading_set(i));cos(proj_heading_set(i))];
    t_r = [cos(proj_heading_set(i));sin(proj_heading_set(i))];
    %近似认为dkr/ds 为0 简化计算
    l_dot2_set(i) = a_h'*n_r - proj_kappa_set(i) * (1 - proj_kappa_set(i) * l_set(i)) * s_dot_set(i)^2;
    s_dot2_set(i) = (1/(1 - proj_kappa_set(i) * l_set(i)))* (a_h' * t_r + 2 * proj_kappa_set(i) * dl_set(i) * s_dot_set(i)^2);
    % 要考虑加速度为0的情况
    if (s_dot2_set(i) < 1e-6)
        ddl_set(i) = 0;
    else
        ddl_set(i) = (l_dot2_set(i) - dl_set(i)*s_dot2_set(i))/(s_dot_set(i)^2);
    end
end

== matlab function EMPlanner_850_155633_cs/Audi_A8_Sedan_1/decision&planning module/EM Planner/obs/obs filter ==
  data: host_x input; obs_x_set_final output; host_y input; host_heading_xy input; obs_x_set_gcs input; obs_y_set_gcs input; obs_velocity_set_gcs input; obs_heading_set_gcs input; obs_y_set_final output; obs_velocity_set_final output; obs_heading_set_final output
function [obs_x_set_final,obs_y_set_final,obs_velocity_set_final,obs_heading_set_final] = fcn(host_x,host_y,host_heading_xy,obs_x_set_gcs,obs_y_set_gcs,obs_velocity_set_gcs,obs_heading_set_gcs)
% 该函数将筛选障碍物，纵向[-10,60] 横向[-10,10]的障碍物才会被考虑
% 该函数只是一种单车道的临时办法，考虑到多车道情况，即使障碍物距离较远也应该考虑
% EM Planner完全体是多车道并行计算的，每个车道都生成参考线然后并行计算出多条轨迹，再选择最优的轨迹作为输出

%传感器最多可以识别32个障碍物
n = 32;
%输出初始化
obs_x_set_final = ones(n,1)*nan;
obs_y_set_final = ones(n,1)*nan;
obs_velocity_set_final = ones(n,1)*nan;
obs_heading_set_final = ones(n,1)*nan;
count = 1;
for i = 1:length(obs_x_set_gcs)
    if isnan(obs_x_set_gcs(i))
        break;
    end
    %自车的heading的方向向量与法向量
    tor = [cos(host_heading_xy);sin(host_heading_xy)];
    nor = [-sin(host_heading_xy);cos(host_heading_xy)];
    %障碍物与自车的距离向量
    vector_obs = [obs_x_set_gcs(i);obs_y_set_gcs(i)] - [host_x;host_y];
    %障碍物纵向距离
    lon_distance = vector_obs'*tor;
    %障碍物横向距离
    lat_distance = vector_obs'*nor;
    
    if (lon_distance < 60) && (lon_distance > -10) && (lat_distance > -25) && (lat_distance < 25)
        obs_x_set_final(count) = obs_x_set_gcs(i);
        obs_y_set_final(count) = obs_y_set_gcs(i);
        obs_heading_set_final(count) = obs_heading_set_gcs(i);
        obs_velocity_set_final(count) = obs_velocity_set_gcs(i);
        count = count + 1;
    end
end

== matlab function EMPlanner_850_155633_cs/Audi_A8_Sedan_1/decision&planning module/EM Planner/MATLAB Function ==
  data: trajectory_heading_final input; y output
function y = fcn(trajectory_heading_final)
y = zeros(421,1);
y(1) = trajectory_heading_final(1);
for i = 2:421
    y(i) = y(i-1) + sin(trajectory_heading_final(i) - trajectory_heading_final(i-1));
end

== matlab function EMPlanner_850_155633_cs/Audi_A8_Sedan_1/decision&planning module/EM Planner/obs/Cartesian2Frenet1/MATLAB Function ==
  data: x_set input; s_set output; y_set input; frenet_path_x input; frenet_path_y input; proj_x_set input; proj_y_set input; proj_heading_set input; proj_match_point_index_set input; index2s input; l_set output
function [s_set,l_set] = fcn(x_set,y_set,frenet_path_x,frenet_path_y,...
    proj_x_set,proj_y_set,proj_heading_set,proj_match_point_index_set,index2s)
    %该函数将计算世界坐标系下的x_set，y_set上的点在frenet_path下的坐标s l
    %输入 x_set,y_set 待坐标转换的点
    %     frenet_path_x,frenet_path_y   frenet坐标轴
    %     proj_x,y,heading,kappa,proj_match_point_index 待坐标转换的点的投影点的信息
    %     index2s   frenet_path的index与s的转换表

    % 由于不知道有多少个点需要做坐标转换，所以需要做缓冲
    n = 128;%最多处理128个点
    %输出初始化
    s_set = ones(n,1)*nan;
    l_set = ones(n,1)*nan;
    for i = 1:length(x_set)
        if isnan(x_set(i))
            break;
        end
        %计算s，写个子函数
        s_set(i) = CalcSFromIndex2S(index2s,frenet_path_x,frenet_path_y,proj_x_set(i),proj_y_set(i),...
            proj_match_point_index_set(i));
        n_r = [-sin(proj_heading_set(i));cos(proj_heading_set(i))];
        r_h = [x_set(i);y_set(i)];
        r_r = [proj_x_set(i);proj_y_set(i)];
        l_set(i) = (r_h - r_r)'*n_r;
    end
end

function s = CalcSFromIndex2S(index2s,path_x,path_y,proj_x,proj_y,proj_match_point_index)
  %该函数将计算当指定index2s的映射关系后，计算点proj_x,proj_y的弧长
  vector_1 = [proj_x;proj_y] - [path_x(proj_match_point_index);path_y(proj_match_point_index)];
  %这里要考虑的更全面一些，因为要考虑到proj_match_point_index有可能在path的起点或终点
  if (proj_match_point_index < length(path_x))
      vector_2 = [path_x(proj_match_point_index + 1);path_y(proj_match_point_index + 1)] - ...
          [path_x(proj_match_point_index);path_y(proj_match_point_index)];
  else
      vector_2 = [path_x(proj_match_point_index);path_y(proj_match_point_index)] - ...
          [path_x(proj_match_point_index - 1);path_y(proj_match_point_index - 1)];
  end
  
  if vector_1'*vector_2 > 0
      s = index2s(proj_match_point_index) + sqrt(vector_1'*vector_1);
  else
      s = index2s(proj_match_point_index) - sqrt(vector_1'*vector_1);
  end
  
  
end

== matlab function EMPlanner_850_155633_cs/Audi_A8_Sedan_1/decision&planning module/EM Planner/obs/Cartesian2Frenet1/MATLAB Function1 ==
  data: l_set input; s_dot_set output; vx_set input; vy_set input; proj_heading_set input; proj_kappa_set input; l_dot_set output; dl_set output
function [s_dot_set,l_dot_set,dl_set] = fcn(l_set,vx_set,vy_set,proj_heading_set,proj_kappa_set)
%该函数将计算frenet坐标系下的s_dot, l_dot, dl/ds
n = 128;
% 输出初始化
s_dot_set = ones(n,1)*nan;
l_dot_set = ones(n,1)*nan;
dl_set = ones(n,1)*nan;

for i = 1 : length(l_set)
    if isnan(l_set(i))
        break;
    end
    v_h = [vx_set(i);vy_set(i)];
    n_r = [-sin(proj_heading_set(i));cos(proj_heading_set(i))];
    t_r = [cos(proj_heading_set(i));sin(proj_heading_set(i))];
    l_dot_set(i) = v_h'*n_r;
    s_dot_set(i) = v_h'*t_r/(1 - proj_kappa_set(i)*l_set(i));
    %%%向量法做cartesian与frenet的转换要更简单，但是也有缺点，向量法必须依赖速度加速度
    %l' = l_dot/s_dot 但是如果s_dot = 0 此方法就失效了
    if abs(s_dot_set(i)) < 1e-6
        dl_set(i) = 0;
    else
        dl_set(i) = l_dot_set(i)/s_dot_set(i);
    end
end

== matlab function EMPlanner_850_155633_cs/Audi_A8_Sedan_2/PathFollower_Preview_1/LateralController/CTRL REFERENCES/Calculate Lateral Error/eml_find_10k_lateral_error_points ==
  data: pvp input size=2; dist_psvehicle output size=10; TrajOffset_x_y_Y input size=3; ActorOffset_Left_Right input; p0 input size=2; PreviewDistance input size=10; Traj_x parameter; Traj_y parameter; Traj_t parameter; Traj_v parameter; RefreshCounter parameter
function dist_psvehicle  = eml_find_10k_lateral_error_points(pvp,TrajOffset_x_y_Y,ActorOffset_Left_Right,p0,PreviewDistance,Traj_x,Traj_y,Traj_t,Traj_v,RefreshCounter)

dist_psvehicle = emlfcn_find_10k_lateral_error_points(pvp,TrajOffset_x_y_Y,ActorOffset_Left_Right,p0,PreviewDistance,Traj_x,Traj_y,Traj_t,Traj_v,RefreshCounter);

% end function

== matlab function EMPlanner_850_155633_cs/Audi_A8_Sedan_1/decision&planning module/EM Planner/obs/Cartesian2Frenet1/MATLAB Function2 ==
  data: ax_set input; s_dot2_set output; ay_set input; proj_heading_set input; proj_kappa_set input; l_set input; s_dot_set input; dl_set input; l_dot2_set output; ddl_set output
function [s_dot2_set,l_dot2_set,ddl_set] = fcn(ax_set,ay_set,proj_heading_set,proj_kappa_set,l_set,s_dot_set,dl_set)
%由于不知道有多少个点需要做坐标转换，设一个最大值做缓冲
n = 128;
% 输出初始化
s_dot2_set = ones(n,1)*nan;
l_dot2_set = ones(n,1)*nan;
ddl_set = ones(n,1)*nan;

for i = 1:length(l_set)
    if isnan(l_set(i))
       break;
    end
    a_h = [ax_set(i);ay_set(i)];
    n_r = [-sin(proj_heading_set(i));cos(proj_heading_set(i))];
    t_r = [cos(proj_heading_set(i));sin(proj_heading_set(i)];
    %近似认为dkr/ds 为0 简化计算
    l_dot2_set(i) = a_h'*n_r - proj_kappa_set(i) * (1 - proj_kappa_set(i) * l_set(i)) * s_dot_set(i)^2;
    s_dot2_set(i) = (1/(1 - proj_kappa_set(i) * l_set(i)))* (a_h' * t_r + 2 * proj_kappa_set(i) * dl_set(i) * s_dot_set(i)^2);
    % 要考虑加速度为0的情况
    if (s_dot2_set(i) < 1e-6)
        ddl_set(i) = 0;
    else
        ddl_set(i) = (l_dot2_set(i) - dl_set(i)*s_dot2_set(i))/(s_dot_set(i)^2);
    end
end

== matlab function EMPlanner_850_155633_cs/Audi_A8_Sedan_1/decision&planning module/EM Planner/obs/MATLAB Function ==
  data: obs_x_set_gcs input; static_obs_x_set output; obs_y_set_gcs input; obs_heading_set_gcs input; obs_velocity_set_gcs input; static_obs_y_set output; dynamic_obs_x_set output; dynamic_obs_y_set output; dynamic_obs_vx_set output; dynamic_obs_vy_set output
function [static_obs_x_set,static_obs_y_set,dynamic_obs_x_set,dynamic_obs_y_set,dynamic_obs_vx_set,dynamic_obs_vy_set]...
    = fcn(obs_x_set_gcs,obs_y_set_gcs,obs_heading_set_gcs,obs_velocity_set_gcs)

%该函数将分类静态障碍物和动态障碍物
%输出初始化
n = 32;
static_obs_x_set = ones(n,1)*nan;
static_obs_y_set = ones(n,1)*nan;
dynamic_obs_x_set = ones(n,1)*nan;
dynamic_obs_y_set = ones(n,1)*nan;
dynamic_obs_vx_set = ones(n,1)*nan;
dynamic_obs_vy_set = ones(n,1)*nan;
count_static = 1;
count_dynamic = 1;
for i = 1:length(obs_x_set_gcs)
    if isnan(obs_velocity_set_gcs(i))
        break;
    end
    if abs(obs_velocity_set_gcs(i)) < 0.1
        static_obs_x_set(count_static) = obs_x_set_gcs(i);
        static_obs_y_set(count_static) = obs_y_set_gcs(i);
        count_static = count_static + 1;
    else
        dynamic_obs_x_set(count_dynamic) = obs_x_set_gcs(i);
        dynamic_obs_y_set(count_dynamic) = obs_y_set_gcs(i);
        dynamic_obs_vx_set(count_dynamic) = obs_velocity_set_gcs(i)*cos(obs_heading_set_gcs(i));
        dynamic_obs_vy_set(count_dynamic) = obs_velocity_set_gcs(i)*sin(obs_heading_set_gcs(i));
        count_dynamic = count_dynamic + 1;      
    end
end

== matlab function EMPlanner_850_155633_cs/Audi_A8_Sedan_1/decision&planning module/EM Planner/calc path length and map between point and s ==
  data: trajectory_x input; path_s_end output; trajectory_y input; path_index2s output
function [path_s_end,path_index2s] = fcn(trajectory_x,trajectory_y)
% 该函数将计算以trajectory的s 与 x y 的对应关系，可以看作是trajectory index2s
n = length(trajectory_x);
path_index2s = zeros(n,1);
sum = 0;
for i = 2:length(trajectory_x)
    if isnan(trajectory_x(i))
        break;
    end
    sum = sum + sqrt((trajectory_x(i) - trajectory_x(i-1))^2 + (trajectory_y(i) - trajectory_y(i-1))^2);
    path_index2s(i) = sum;
end
% 计算出trajectory的长度
if i == n
    path_s_end = path_index2s(end);
else
    % 因为循环的退出条件为isnan(trajectory_x(i)) 所以 i 所对应的数为 nan 
    path_s_end = path_index2s(i - 1);
end
